simulink model "Linear_Model_Ters_Sarkac"  (R2022a)
settings: Solver=ode4  StartTime=0.0  StopTime=10.0  FixedStep=1/1000  RelTol=1e-3
InitFcn:
  | Sarkac_Parametrelerini_Yukle
values from neighbouring files (symbols this model uses):
  A = [0      1              0           0 ... (first row only)    [Sarkac_Parametrelerini_Yukle.m]
  B = [     0 ... (first row only)    [Sarkac_Parametrelerini_Yukle.m]
  Baslangic_Degerleri_Lin = [0,0,0,0]    [Sarkac_Parametrelerini_Yukle.m]
  C = [1 0 0 0 ... (first row only)    [Sarkac_Parametrelerini_Yukle.m]
  D = [0 ... (first row only)    [Sarkac_Parametrelerini_Yukle.m]
undefined symbols (not defined in the file or in its folder): sigbuilder_block
libraries: vrlib x1
settings Model: Creator=Fatabi  LastModifiedBy=Fatabi
settings SolverCC: AlgebraicLoopSolver=TrustRegion
settings DebuggingCC: UnconnectedInputMsg=warning  UnconnectedOutputMsg=warning  UnconnectedLineMsg=warning  SFMachineParentedDataDiag=warning

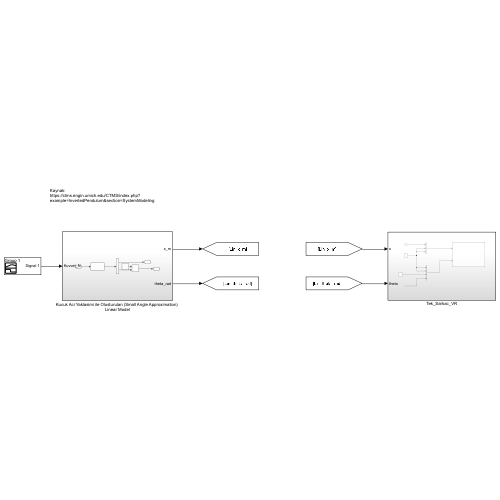
[thumbnail: Simulink's stored preview of the top-level diagram]
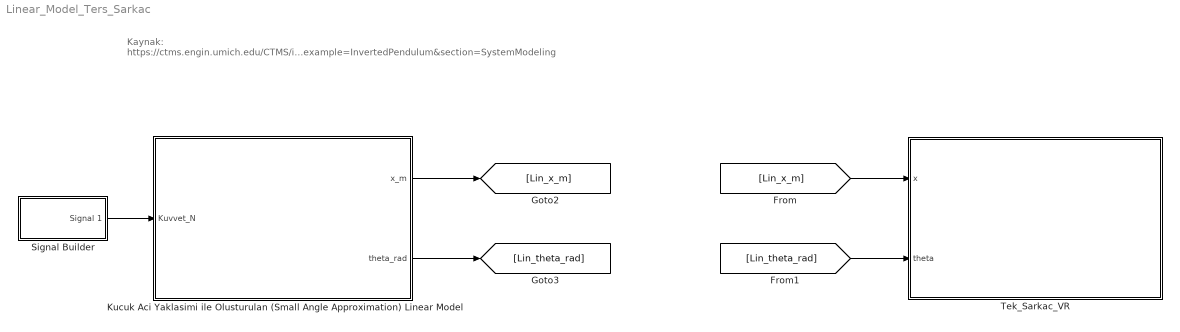
== system Linear_Model_Ters_Sarkac ==
  note: Kaynak:
      | https://ctms.engin.umich.edu/CTMS/index.php?example=InvertedPendulum&section=SystemModeling
  Kucuk Aci Yaklasimi ile Olusturulan (Small Angle Approximation) Linear Model : Subsystem
  Signal Builder : Subsystem  Tag=STV Subsys  LoadFcn=sigbuilder_block('load');  StartFcn=sigbuilder_block('start');  StopFcn=sigbuilder_block('stop');  ClipboardFcn=sigbuilder_block('clipboard');  mask(Sigbuilder block){tuvar=[0:10]}
      mask help: Simulink:masks:SigbuilderBlock_MD
      mask init:
      | if ~strcmp(get_param(bdroot(gcbh),'SimulationStatus'),'stopped') tuvar = sigbuilder_block('maskInit'); end
      settings: CopyFcn=sigbuilder_block('copy');  DeleteFcn=sigbuilder_block('delete');  ModelCloseFcn=sigbuilder_block('modelClose');  PreSaveFcn=sigbuilder_block('preSave');  PauseFcn=sigbuilder_block('pause');  ContinueFcn=sigbuilder_block('continue');  NameChangeFcn=sigbuilder_block('namechange');  OpenFcn=sigbuilder_block('open',[338.25 225.75 550.5 399.75 ]);  CloseFcn=sigbuilder_block('close');
      mask Display: plot(0, 0, 100, 100,[2, 2, 32, 32, 2], [68, 8, 8, 68, 68],[32, 2], [38, 38], [32, 19, 2],[53, 60, 44], [32, 17, 17, 2],[16, 16, 31, 31]);txt = getActiveGroup(gcbh);text(2, 100, txt,'verticalAlignment', 'top');
  "Tek_Sarkac_VR " : Subsystem
  wires:
  Signal Builder/1(Signal 1) -> Kucuk Aci Yaklasimi ile Olusturulan (Small Angle Approximation) Linear Model/1(Kuvvet_N)
  Kucuk Aci Yaklasimi ile Olusturulan (Small Angle Approximation) Linear Model/1(x_m) -> [Lin_x_m]
  Kucuk Aci Yaklasimi ile Olusturulan (Small Angle Approximation) Linear Model/2(theta_rad) -> [Lin_theta_rad]
  [Lin_x_m] -> "Tek_Sarkac_VR "/1(x)
  [Lin_theta_rad] -> "Tek_Sarkac_VR "/2("theta ")

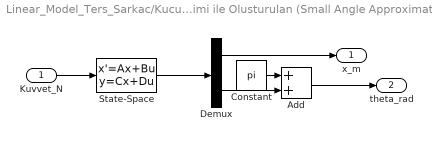
== system Linear_Model_Ters_Sarkac/Kucuk Aci Yaklasimi ile Olusturulan (Small Angle Approximation) Linear Model ==
  Kuvvet_N : Inport
  Add : Sum
  Constant : Constant  Value=pi
  Demux : Demux  Outputs=2
  State-Space : StateSpace  A=A  B=B  C=C  D=D  InitialCondition=Baslangic_Degerleri_Lin
  x_m : Outport
  theta_rad : Outport  Port=2
  wires:
  State-Space/1 -> Demux/1
  Demux/1 -> x_m/1
  Demux/2 -> Add/2
  Kuvvet_N/1 -> State-Space/1
  Add/1 -> theta_rad/1
  Constant/1 -> Add/1

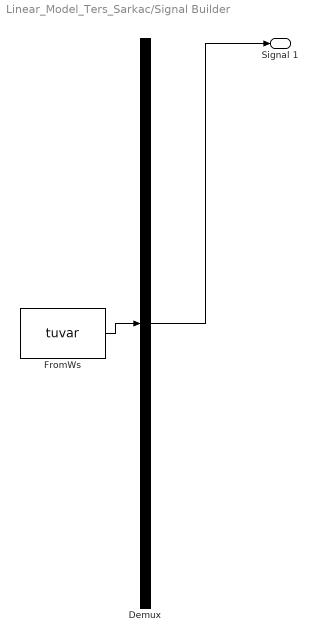
== system Linear_Model_Ters_Sarkac/Signal Builder ==
  Demux : Demux  Tag=STV Demux  Outputs=1
      settings: DisplayOption=none
  FromWs : FromWorkspace  Tag=STV FromWs  VariableName=tuvar
      SigBuilderData=|
      | common.afterFinalStr = 'Extrapolate'
      | common.sampleTime = 0
      | dataSet.timeRange = [0 10]
      | dataSet.name = 'Group 1'
      | sbobj.Groups.Name = 'Group 1'
      | sbobj.Groups.Signals.Name = 'Signal 1'
      | sbobj.Groups.Signals.XData = [0 1 1 1.5 1.5 10]
      | sbobj.Groups.Signals.YData = [0 0 1 1 0 0]
  Signal 1 : Outport  Tag=STV Outport
  wires:
  Demux/1 -> Signal 1/1
  FromWs/1 -> Demux/1

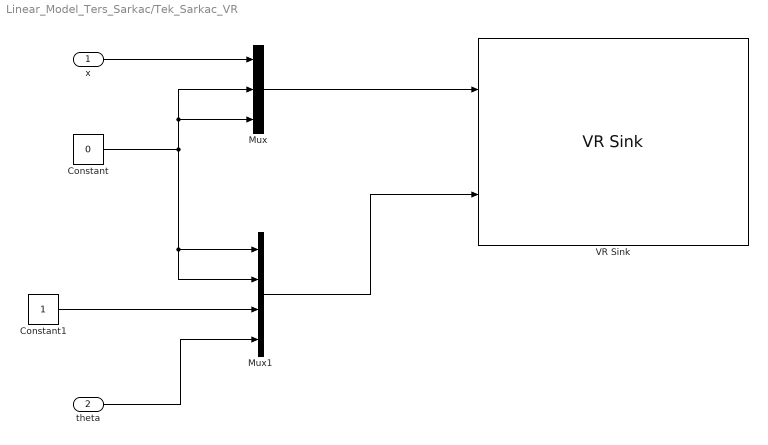
== system Linear_Model_Ters_Sarkac/Tek_Sarkac_VR  ==
  x : Inport
  "theta " : Inport  Port=2
  Constant : Constant  Value=0
  Constant1 : Constant
  Mux : Mux  Inputs=3
  Mux1 : Mux
  VR Sink : vrlib/VR Sink  InstantiateOnLoad=on  SampleTime=0.02  ViewEnable=on  RemoteChange=off  RemoteView=off  FieldsWritten=Kutu.translation.3.1.1.double#Mentese1.rotation.4.1.1.double  WorldFileName=sarkac.wrl  AutoView=off  VideoDimensions=[]  AllowVariableSize=off
  wires:
  x/1 -> Mux/1
  Constant/1 -> Mux/3, Mux/2, Mux1/2, Mux1/1
  "theta "/1 -> Mux1/4
  Constant1/1 -> Mux1/3
  Mux/1 -> VR Sink/1
  Mux1/1 -> VR Sink/2
